simulink model "a4_quan_control_ekf_estimate"  (R2018b)
settings: Solver=VariableStepAuto  StartTime=0.0  StopTime=5  RelTol=0.1
undefined symbols (not defined in the file or in its folder): AngularState, Attitude, AttitudeController, DifferentialFlat, drawQuad, EKFState, InverseMapping, LQRController, P, Sensor, StateEstimate, Trajectory
settings Model: Creator=erics  LastModifiedBy=erics

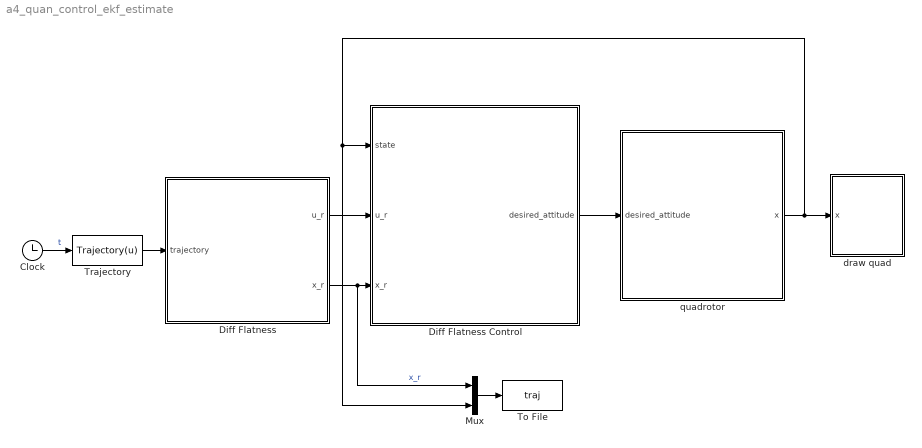
== system a4_quan_control_ekf_estimate ==
  Clock : Clock
  Diff Flatness : Subsystem
  Diff Flatness Control : Subsystem
  Mux : Mux  Inputs=2
  To File : ToFile  Filename=traj  MatrixName=Xt  SaveFormat=Timeseries
  "Trajectory " : MATLABFcn  MATLABFcn=Trajectory(u)  OutputDimensions=12
  draw quad : Subsystem
      mask init:
      | P.courselength = 11;
      | P.coursewidth = 6;
      |     %6ft columns plus four feet of head room
      | P.courseheight = 10;
      | 
      | % quadrotor starting point at 3 ft high and 3 ft in front of the pillars 
      | P.zstart = 0;
      | P.xstart = 0;
      | P.ystart = 0;
      | 
      | % quadrotor dimentions
      |     %2 inches from the center
      | P.boxlength = 1/6;
      | P.boxwidth = P.boxlength;
      |     %4.5 inches from the bottom to the top
      | P.boxheight = 0.375;
      |     %6 inches from box to motor
      | P.armlength = 0.5;
      |     %1/8 inch from center to the side of a rod
      | P.armwidth = 1/96;
      |     %1/4 inch from the top of the box
      | P.armposition = 1/48;
      |     %25*(2)^(1/2)/2 inches from center to perimeter along x and y axis
      | P.perimeter = 1.47;
      |     %perimeter has 3/16 inch width
      | P.periwidth = 1/64;
      | 
      | % pillar dimentions
      |     %6 ft high
      | P.pillarheight = 6;
      |     %5 ft offset;
      | P.pillarposition = 5; 
      |     %5 in radius
      | P.pillarradius = 0.417;
      |     %The adjustment for the none circular pillar
      | P.pillaradd = 0.167;
      |     %The height of each strip on color
      | P.pillarc1 = 0.833; 
      | P.pillarc2 = 0.5;
      mask Display: image(imread('tv.jpg'))
  quadrotor : Subsystem
  wires:
  Clock/1 -> "Trajectory "/1  "t"
  quadrotor/1(x) -> draw quad/1(x), Diff Flatness Control/1(state), Mux/2
  Diff Flatness Control/1(desired_attitude) -> quadrotor/1(desired_attitude)
  "Trajectory "/1 -> Diff Flatness/1(trajectory)
  Diff Flatness/1(u_r) -> Diff Flatness Control/2(u_r)
  Diff Flatness/2(x_r) -> Mux/1, Diff Flatness Control/3(x_r)  "x_r"
  Mux/1 -> To File/1

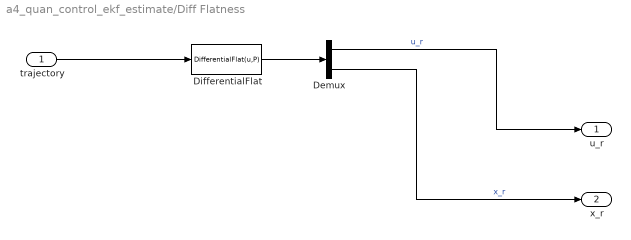
== system a4_quan_control_ekf_estimate/Diff Flatness ==
  trajectory : Inport
  Demux : Demux  Outputs=[4,-1]
  DifferentialFlat : MATLABFcn  MATLABFcn=DifferentialFlat(u,P)  OutputDimensions=11
  u_r : Outport
  x_r : Outport  Port=2
  wires:
  DifferentialFlat/1 -> Demux/1
  Demux/1 -> u_r/1  "u_r"
  trajectory/1 -> DifferentialFlat/1
  Demux/2 -> x_r/1  "x_r"

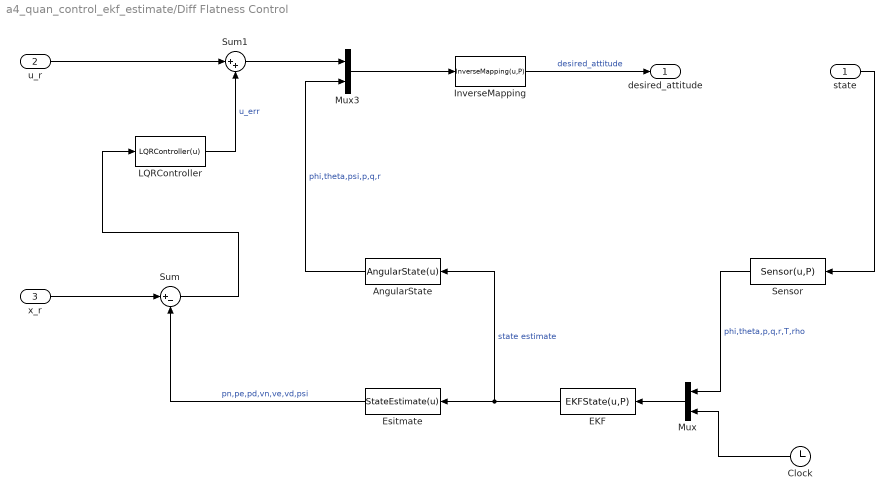
== system a4_quan_control_ekf_estimate/Diff Flatness Control ==
  state : Inport
  u_r : Inport  Port=2
  x_r : Inport  Port=3
  AngularState : MATLABFcn  MATLABFcn=AngularState(u)  OutputDimensions=6
  Clock : Clock
  EKF : MATLABFcn  MATLABFcn=EKFState(u,P)  OutputDimensions=12
  Esitmate : MATLABFcn  MATLABFcn=StateEstimate(u)  OutputDimensions=7
  InverseMapping : MATLABFcn  MATLABFcn=InverseMapping(u,P)  OutputDimensions=4
  LQRController : MATLABFcn  MATLABFcn=LQRController(u)  OutputDimensions=4  Output1D=off
  Mux : Mux  Inputs=2
  Mux3 : Mux  Inputs=2
  Sensor : MATLABFcn  MATLABFcn=Sensor(u,P)
  Sum : Sum  Inputs=|+-
  Sum1 : Sum  Inputs=|++
  desired_attitude : Outport
  wires:
  x_r/1 -> Sum/1
  LQRController/1 -> Sum1/2  "u_err"
  u_r/1 -> Sum1/1
  Mux3/1 -> InverseMapping/1
  Sum1/1 -> Mux3/1
  InverseMapping/1 -> desired_attitude/1  "desired_attitude"
  Sum/1 -> LQRController/1
  state/1 -> Sensor/1
  Esitmate/1 -> Sum/2  "pn,pe,pd,vn,ve,vd,psi"
  EKF/1 -> AngularState/1, Esitmate/1  "state estimate"
  AngularState/1 -> Mux3/2  "phi,theta,psi,p,q,r"
  Sensor/1 -> Mux/1  "phi,theta,p,q,r,T,rho"
  Clock/1 -> Mux/2
  Mux/1 -> EKF/1

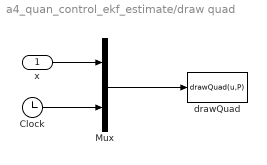
== system a4_quan_control_ekf_estimate/draw quad ==
  x : Inport
  Clock : Clock
  Mux : Mux  Inputs=2
  drawQuad : MATLABFcn  MATLABFcn=drawQuad(u,P)  OutputDimensions=0  SampleTime=0.1
  wires:
  Mux/1 -> drawQuad/1
  x/1 -> Mux/1
  Clock/1 -> Mux/2

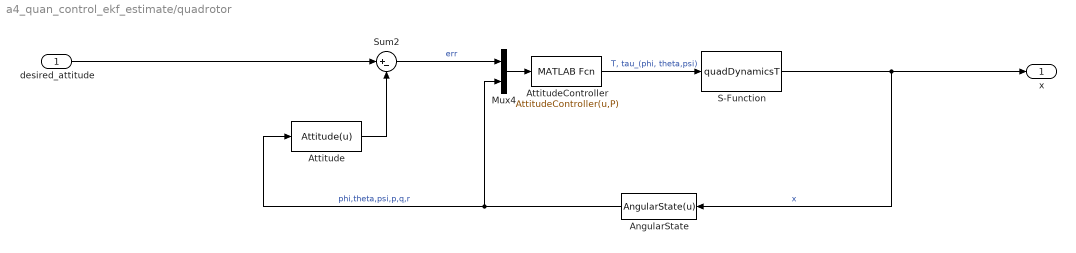
== system a4_quan_control_ekf_estimate/quadrotor ==
  desired_attitude : Inport
  AngularState : MATLABFcn  MATLABFcn=AngularState(u)  OutputDimensions=6
  Attitude : MATLABFcn  MATLABFcn=Attitude(u)  OutputDimensions=4
  AttitudeController : MATLABFcn  MATLABFcn=AttitudeController(u,P)  OutputDimensions=4
  Mux4 : Mux  Inputs=2
  S-Function : S-Function  FunctionName=quadDynamicsT  Parameters=P  SFunctionDeploymentMode=off  EnableBusSupport=off
  Sum2 : Sum  Inputs=|+-
  x : Outport
  wires:
  S-Function/1 -> x/1, AngularState/1  "x"
  Mux4/1 -> AttitudeController/1
  Attitude/1 -> Sum2/2
  AngularState/1 -> Attitude/1, Mux4/2  "phi,theta,psi,p,q,r"
  desired_attitude/1 -> Sum2/1
  AttitudeController/1 -> S-Function/1  "T, tau_(phi, theta,psi)"
  Sum2/1 -> Mux4/1  "err"
